simulink model "mimo2"  (Simulink 3.00)
settings: Solver=ode45  SolverMode=SingleTasking  StartTime=0.0  StopTime=50  MaxStep=0.010  RelTol=1e-3  AbsTol=1e-3
settings Model: TimeSaveName=t  SaveOutput=off

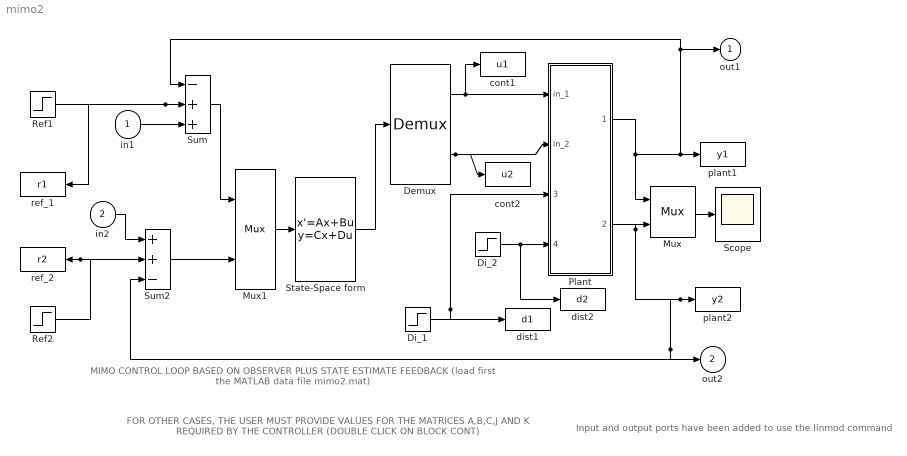
== system mimo2 ==
  note: FOR OTHER CASES, THE USER MUST PROVIDE VALUES FOR THE MATRICES A,B,C,J AND K
      | REQUIRED BY THE CONTROLLER (DOUBLE CLICK ON BLOCK CONT)
  note: MIMO CONTROL LOOP BASED ON OBSERVER PLUS STATE ESTIMATE FEEDBACK
      | (load first the MATLAB data file mimo2.mat)
  note: Input and output ports
      | have been added
      | to use the linmod command
  in1 : Inport  Port=1  PortWidth=-1  SampleTime=-1  DataType=auto
      settings: SignalType=auto
  in2 : Inport  Port=2  PortWidth=-1  SampleTime=-1  DataType=auto
      settings: SignalType=auto
  Demux : Demux  Outputs=2
  Di_1 : Step  Time=20  Before=0  After=1  SampleTime=0
  Di_2 : Step  Time=30  Before=0  After=-1  SampleTime=0
  Mux : Mux  Inputs=2
      settings: DisplayOption=none
  Mux1 : Mux  Inputs=2
      settings: DisplayOption=none
  Plant : Subsystem
      mask Type: PLANT
      mask Display: disp('Plant')
  Ref1 : Step  Time=1  Before=0  After=1  SampleTime=0
  Ref2 : Step  Time=10  Before=0  After=-1  SampleTime=0
  Scope : Scope
      settings: TickLabels=on  TimeRange=50.000000  YMin=-2  YMax=2  SaveToWorkspace=off  SaveName=ScopeData  DataFormat=Matrix
  State-Space form : StateSpace  A=A-J*C-B*K  B=J  C=K  D=0*(B'*B)  X0=0  mask(Controller block){@1=A, @2=B, @3=C, @4=J, @5=K}
      mask prompts: @1 "matrix A:"; @2 "matrix B:"; @3 "matrix C:"; @4 "observer gain matrix J:"; @5 "feedback gain matrix K:"
      mask help: Controller
      mask init:
      | A=@1;B=@2;C=@3;J=@4;K=@5
      mask Help: This controller is implemented as shown in section 11.5, in Princicples of Control Design
      mask Display: disp('CONT')
  Sum : Sum  Inputs=-++  SaturateOnIntegerOverflow=on
  Sum2 : Sum  Inputs=++-  SaturateOnIntegerOverflow=on
  cont1 : ToWorkspace  VariableName=u1  SampleTime=0  SaveFormat=Matrix
      settings: Buffer=10000
  cont2 : ToWorkspace  VariableName=u2  SampleTime=0  SaveFormat=Matrix
      settings: Buffer=10000
  dist1 : ToWorkspace  VariableName=d1  SampleTime=0  SaveFormat=Matrix
      settings: Buffer=10000
  dist2 : ToWorkspace  VariableName=d2  SampleTime=0  SaveFormat=Matrix
      settings: Buffer=10000
  plant1 : ToWorkspace  VariableName=y1  SampleTime=0  SaveFormat=Matrix
      settings: Buffer=10000
  plant2 : ToWorkspace  VariableName=y2  SampleTime=0  SaveFormat=Matrix
      settings: Buffer=10000
  ref_1 : ToWorkspace  VariableName=r1  SampleTime=0  SaveFormat=Matrix
      settings: Buffer=10000
  ref_2 : ToWorkspace  VariableName=r2  SampleTime=0  SaveFormat=Matrix
      settings: Buffer=10000
  out1 : Outport  Port=1  InitialOutput=0
  out2 : Outport  Port=2  InitialOutput=0
  wires:
  Mux/1 -> Scope/1
  Plant/2(out_2) -> Mux/2, plant2/1, Sum2/3, out2/1
  Plant/1(out_1) -> Mux/1, plant1/1, Sum/1, out1/1
  Sum2/1 -> Mux1/2
  in1/1 -> Sum/3
  Sum/1 -> Mux1/1
  Ref1/1 -> Sum/2, ref_1/1
  Mux1/1 -> State-Space form/1
  State-Space form/1 -> Demux/1
  in2/1 -> Sum2/1
  Ref2/1 -> ref_2/1, Sum2/2
  Di_1/1 -> dist1/1, Plant/3(Inport)
  Demux/2 -> Plant/2(in_2), cont2/1
  Demux/1 -> Plant/1(in_1), cont1/1
  Di_2/1 -> Plant/4(Inport1), dist2/1

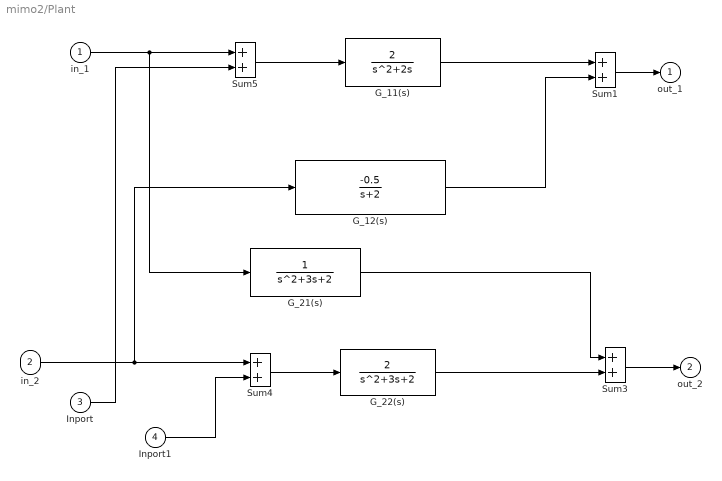
== system mimo2/Plant ==
  in_1 : Inport  Port=1  PortWidth=-1  SampleTime=-1  DataType=auto
      settings: SignalType=auto
  in_2 : Inport  Port=2  PortWidth=-1  SampleTime=-1  DataType=auto
      settings: SignalType=auto
  Inport : Inport  Port=3  PortWidth=-1  SampleTime=-1  DataType=auto
      settings: SignalType=auto
  Inport1 : Inport  Port=4  PortWidth=-1  SampleTime=-1  DataType=auto
      settings: SignalType=auto
  G_11(s) : TransferFcn  Numerator=2  Denominator=[1 2 0]
  G_12(s) : TransferFcn  Numerator=-0.5  Denominator="[1  2  ]"
  G_21(s) : TransferFcn  Numerator=1  Denominator=[1 3 2]
  G_22(s) : TransferFcn  Numerator=2  Denominator=[1 3 2]
  Sum{1,3..5} (4 alike) : Sum  Inputs=++  SaturateOnIntegerOverflow=on
  out_1 : Outport  Port=1  InitialOutput=0
  out_2 : Outport  Port=2  InitialOutput=0
  wires:
  G_11(s)/1 -> Sum1/1
  Sum1/1 -> out_1/1
  G_12(s)/1 -> Sum1/2
  Sum5/1 -> G_11(s)/1
  in_1/1 -> Sum5/1, G_21(s)/1
  G_21(s)/1 -> Sum3/1
  Sum3/1 -> out_2/1
  Sum4/1 -> G_22(s)/1
  G_22(s)/1 -> Sum3/2
  Inport1/1 -> Sum4/2
  in_2/1 -> Sum4/1, G_12(s)/1
  Inport/1 -> Sum5/2
